simulink model "FiltroAdaptado"  (R2020b)
settings: Solver=ode45  StartTime=0.0  StopTime=Tb  RelTol=1e-3  EnableMultiTasking=on
values from neighbouring files (symbols this model uses):
  Canal = 600    [filtroadaptado.m]
  Ts = .02+(76/10000)    (= 0.0276)    [filtroadaptado.m]
  valRuido = 12000    [filtroadaptado.m]
libraries: simulink_extras x1, commnoisgen2 x1
settings Model: Creator=Dario  LastModifiedBy=Agustin
settings DataIOCC: LimitDataPoints=on  SaveFormat=Array  ReturnWorkspaceOutputs=off
settings OptimizationCC: LifeSpan=inf
settings DebuggingCC: UnderspecifiedInitializationDetection=Classic  MergeDetectMultiDrivingBlocksExec=none  SolverPrmCheckMsg=warning  StateNameClashWarn=warning  SFUnexpectedBacktrackingDiag=warning  SFNoUnconditionalDefaultTransitionDiag=warning  SFExecutionAtInitializationDiag=none  ArithmeticOperatorsInVariantConditions=warning
settings HardwareCC: ProdBitPerPointer=32  ProdBitPerSizeT=32  ProdBitPerPtrDiffT=32  ProdLargestAtomicFloat=None  ProdIntDivRoundTo=Undefined  ProdEndianess=Unspecified  ProdWordSize=32  ProdHWDeviceType=32-bit Generic
settings ModelReferenceCC: PropagateSignalLabelsOutOfModel=off
settings SFSimCC: SimUseLocalCustomCode=off  CustomCodeUndefinedFunction=UseInterfaceOnly
settings RTWCC: RTWUseLocalCustomCode=off
settings CodeAppCC: StateflowObjectComments=on
settings GRTTargetCC: TargetLangStandard=C89/C90 (ANSI)
settings ConfigComp: CovMetricSettings=dw  CovSaveCumulativeToWorkspaceVar=on  CovSaveSingleToWorkspaceVar=on  CovExternalEMLEnable=off

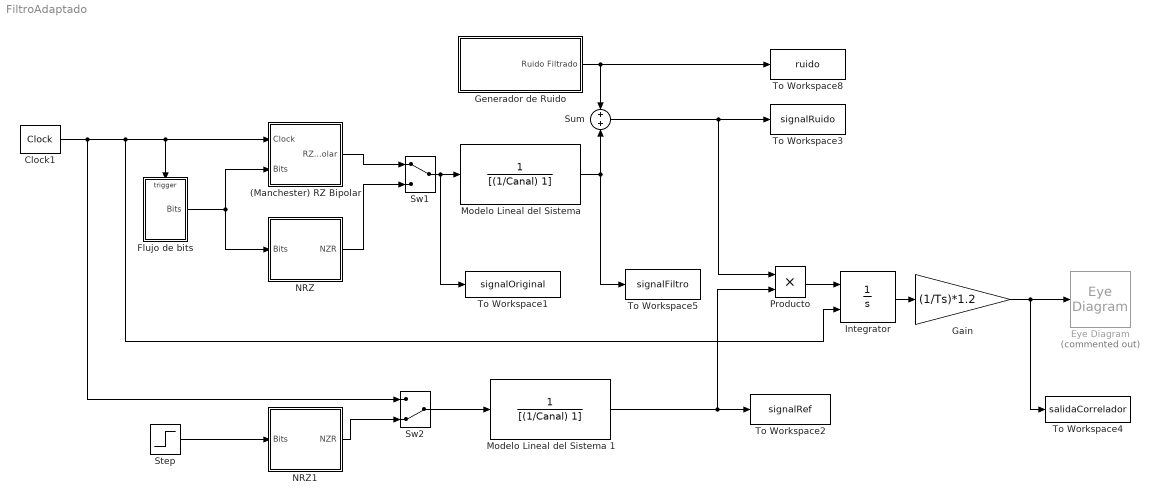
== system FiltroAdaptado ==
  (Manchester) RZ Bipolar : Subsystem
  Clock1 : simulink_extras/Flip Flops/Clock  period=Ts
  Eye Diagram : EyeDiagram  Commented=on
  Flujo de bits : Subsystem
  Gain : Gain  Gain=(1/Ts)*1.2  SampleTime=Ts/500
  Generador de Ruido : Subsystem
  Integrator : Integrator  ExternalReset=rising
  "Modelo Lineal del Sistema " : TransferFcn  Denominator=[(1/Canal) 1]
  Modelo Lineal del Sistema 1 : TransferFcn  Denominator=[(1/Canal) 1]
  NRZ : Subsystem
  NRZ1 : Subsystem
  Producto : Product  RndMeth=Zero
  Step : Step  Time=0  SampleTime=0
  Sum : Sum  Inputs=+|+
  Sw1 : ManualSwitch
  Sw2 : ManualSwitch  CurrentSetting=0
  To Workspace1 : ToWorkspace  VariableName=signalOriginal  SaveFormat=Timeseries  SampleTime=-1
  To Workspace2 : ToWorkspace  VariableName=signalRef  SaveFormat=Timeseries  SampleTime=-1
  To Workspace3 : ToWorkspace  VariableName=signalRuido  SaveFormat=Timeseries  SampleTime=-1
  To Workspace4 : ToWorkspace  VariableName=salidaCorrelador  SaveFormat=Timeseries  SampleTime=-1
  To Workspace5 : ToWorkspace  VariableName=signalFiltro  SaveFormat=Timeseries  SampleTime=-1
  To Workspace8 : ToWorkspace  VariableName=ruido  SaveFormat=Timeseries  SampleTime=-1
  wires:
  Flujo de bits/1(Bits) -> (Manchester) RZ Bipolar/2(Bits), NRZ/1(Bits)
  Sw1/1 -> To Workspace1/1, "Modelo Lineal del Sistema "/1
  Generador de Ruido/1(Ruido Filtrado) -> To Workspace8/1, Sum/1
  Sum/1 -> Producto/1, To Workspace3/1
  Integrator/1 -> Gain/1
  Step/1 -> NRZ1/1(Bits)
  Sw2/1 -> Modelo Lineal del Sistema 1/1
  Producto/1 -> Integrator/1
  Clock1/1 -> (Manchester) RZ Bipolar/1(Clock), Flujo de bits/Trigger, Integrator/2, Sw2/1
  NRZ1/1(NZR) -> Sw2/2
  (Manchester) RZ Bipolar/1(RZ-Bipolar) -> Sw1/1
  NRZ/1(NZR) -> Sw1/2
  Modelo Lineal del Sistema 1/1 -> To Workspace2/1, Producto/2
  Gain/1 -> Eye Diagram/1, To Workspace4/1
  "Modelo Lineal del Sistema "/1 -> Sum/2, To Workspace5/1

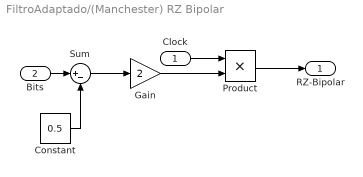
== system FiltroAdaptado/(Manchester) RZ Bipolar ==
  Clock : Inport
  Bits : Inport  Port=2
  Constant : Constant  Value=0.5
  Gain : Gain  Gain=2
  Product : Product  RndMeth=Zero
  Sum : Sum  Inputs=|+-
  RZ-Bipolar : Outport  VectorParamsAs1DForOutWhenUnconnected=off
  wires:
  Constant/1 -> Sum/2
  Sum/1 -> Gain/1
  Gain/1 -> Product/2
  Product/1 -> RZ-Bipolar/1
  Clock/1 -> Product/1
  Bits/1 -> Sum/1

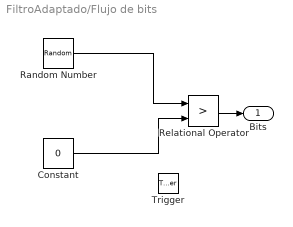
== system FiltroAdaptado/Flujo de bits ==
  Trigger : TriggerPort  VariantControl=Variant
  Constant : Constant  Value=0
  Random Number : RandomNumber  Seed=10
  Relational Operator : RelationalOperator  Operator=>  OutDataTypeStr=boolean  RndMeth=Nearest
  Bits : Outport  VectorParamsAs1DForOutWhenUnconnected=off
  wires:
  Random Number/1 -> Relational Operator/1
  Constant/1 -> Relational Operator/2
  Relational Operator/1 -> Bits/1

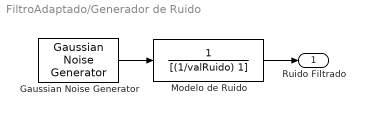
== system FiltroAdaptado/Generador de Ruido ==
  Gaussian Noise Generator : commnoisgen2/Gaussian Noise Generator  m=0  d=varianza  s=41  Ts=0.00001  frameBased=off  sampPerFrame=1  orient=off  outDataType=double
      settings: SourceProductBaseCode=CM
  "Modelo de Ruido    " : TransferFcn  Denominator=[(1/valRuido) 1]
  Ruido Filtrado : Outport  VectorParamsAs1DForOutWhenUnconnected=off
  wires:
  Gaussian Noise Generator/1 -> "Modelo de Ruido    "/1
  "Modelo de Ruido    "/1 -> Ruido Filtrado/1

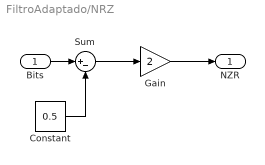
== system FiltroAdaptado/NRZ ==
  Bits : Inport
  Constant : Constant  Value=0.5
  Gain : Gain  Gain=2
  Sum : Sum  Inputs=|+-
  NZR : Outport  VectorParamsAs1DForOutWhenUnconnected=off
  wires:
  Bits/1 -> Sum/1
  Constant/1 -> Sum/2
  Sum/1 -> Gain/1
  Gain/1 -> NZR/1

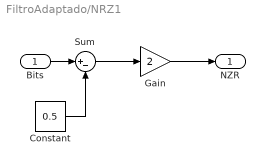
== system FiltroAdaptado/NRZ1 ==
  Bits : Inport
  Constant : Constant  Value=0.5
  Gain : Gain  Gain=2
  Sum : Sum  Inputs=|+-
  NZR : Outport  VectorParamsAs1DForOutWhenUnconnected=off
  wires:
  Bits/1 -> Sum/1
  Constant/1 -> Sum/2
  Sum/1 -> Gain/1
  Gain/1 -> NZR/1
